simulink model "DTNS_SIM2"  (R2022a)
settings: Solver=ode4  StartTime=0.0  StopTime=100  FixedStep=0.01  RelTol=1e-3  EnableMultiTasking=on
PreLoadFcn:
  | listing = dir;
  | if (contains([listing.name], 'MAP')) &&  (contains([listing.name], 'DTNS_SIM.slx'))
  |     addpath('./AGR', './TRN', './TCAF', './FTG', './DYN', './FLCC', './GPS', './RALT', './INS', './MAP');
  |     addpath('./MAP/MAP_DB');
  | else
  |     warning('[DTNS_SIM.slx]는 DTNS 프로젝트 최상단 경로에 위치해야 합니다.');
  | end
  | 
  | load('BUS_STRUCTURE_DYN.mat');
  | load('BUS_STRUCTURE_FLCC.mat');
  | load('BUS_STRUCTURE_RALT.mat');
  | load('BUS_STRUCTURE_INS.mat');
  | load('BUS_STRUCTURE_GPS.mat');
  | load('BusStructureTRN.mat');
  | load('BusStructureLOSR.mat');
  | load('BusStructureHR.mat');
  | load('BusStructureCR.mat');
  | FTG_initState;
InitFcn:
  | listing = dir;
  | if (contains([listing.name], 'MAP')) &&  (contains([listing.name], 'DTNS_SIM.slx'))
  |     addpath('./AGR', './TRN', './TCAF', './FTG', './DYN', './FLCC', './GPS', './RALT', './INS', './MAP');
  |     addpath('./MAP/MAP_DB');
  | else
  |     warning('[DTNS_SIM.slx]는 DTNS 프로젝트 최상단 경로에 위치해야 합니다.');
  | end
  | 
  | load('BUS_STRUCTURE_DYN.mat');
  | load('BUS_STRUCTURE_FLCC.mat');
  | load('BUS_STRUCTURE_RALT.mat');
  | load('BUS_STRUCTURE_INS.mat');
  | load('BUS_STRUCTURE_GPS.mat');
  | load('BusStructureTRN.mat');
  | load('BusStructureLOSR.mat');
  | load('BusStructureHR.mat');
  | load('BusStructureCR.mat');
  | FTG_initState;
libraries: aerolibconvert2 x14, simulink_extras x5
(part 2 of 2)

== matlab function DTNS_SIM2/ControlTFInput ==
  data: inBus input Bus: DTFInput; DTFInput output Bus: DTFInput; RALTDatapumpPrev input
function DTFInput = ControlTFInput(inBus, RALTDatapumpPrev)
%ControlTFInput
persistent time dt
if isempty(time)
    time = 0.0;
end
if isempty(dt)
    dt = 0.01;
end
% -------------------------------------------------------------------------
% CONTROL flag
CONTROL_ACTIVATED = true;

% Copy
DTFInput = inBus;

if CONTROL_ACTIVATED
    % Default
    DTFInput.selected   = SET_VALUE(DTFInput.selected, true, time, 0, inf);
    DTFInput.rideQuality= SET_VALUE(DTFInput.rideQuality, uint16(3), time, 0, inf);
    DTFInput.msd        = SET_VALUE(DTFInput.msd, 500, time, 0, inf);
    DTFInput.raltValid  = SET_VALUE(DTFInput.raltValid, RALTDatapumpPrev.RadarAltitudeValid, time, 0, inf);
    DTFInput.raltAlt    = SET_VALUE(DTFInput.raltAlt, RALTDatapumpPrev.RadarAltitude, time, 0, inf);

    % Control
%     outBus.msd = SET_VALUE(outBus.msd, 500, time, 100, 50);
%     outBus.msd = SET_VALUE(outBus.msd, 500, time, 200, 50);

end

% Update Time
time = time + dt;
end

function out = SET_VALUE(in, value, curTime, triggerTime, duration)
out = in;
if (triggerTime <= curTime) && (curTime <= triggerTime+duration)
    out = value;
else
end
end

== matlab function DTNS_SIM2/TRNDataProcess/Subsystem3/Flag_WoW ==
  data: time input; WeightOnWheels output
function WeightOnWheels  = fcn(time)

% WeightOnWheels
% False[0]_flight / True[1]_ground

% if time <= 30
if time < 0
    WeightOnWheels = boolean(true);
else
    WeightOnWheels = boolean(false);
end

end

== matlab function DTNS_SIM2/TRNDataProcess/Subsystem3/MATLAB Function ==
  data: count input; count output
function count = fcn(count)

count = count + 0.04;

== matlab function DTNS_SIM2/TRNDataProcess/Subsystem3/Subsystem1/MATLAB Function1 ==
  data: WoW input; time input; lat_bias output; lon_bias output
function [lat_bias,lon_bias] = fcn(WoW, time)
%% parameters
lat2m = 111000;
lon2m = 91170;
bias1 = 200;   % 500m
bias2 = 200;   % 500m


%%
% if time > 60
if time >= 0
    if WoW == 0                % 0_flight / 1_ground
        lat_bias = bias1/lat2m;
        lon_bias = bias2/lon2m;
    else
        lat_bias = 0;
        lon_bias = 0;
    end
else
    lat_bias = 0;
    lon_bias = 0;
end

== matlab function DTNS_SIM2/TRNDataProcess/Subsystem3/Subsystem1/MATLAB Function3 ==
  data: u input; a output; b output
function [a,b]  = fcn(u)

% WeightOnWheels
if(u==1)
    a = boolean(true);
    b = boolean(true);
else
    a = boolean(false);
    b = boolean(false);
end

end

== matlab function DTNS_SIM2/Visualize/calcTerrainRoughness ==
  data: lat input; R output; lon input; hDEM output
function [R, hDEM] = calcTerrainRoughness(lat, lon)

lat2m = 110961.7060516;
lon2m = 89476.51124;

d_Lat = 90/lat2m; d_Lon = 90/lon2m;
d = 90;

hDEM = 0.0;
A=0.0; B=0.0; C=0.0; D=0.0; E=0.0; F=0.0; G=0.0; H=0.0; I=0.0; 

A = coder.ceval('MAPGetTerrainHeight', lat+d_Lat, lon-d_Lon);
B = coder.ceval('MAPGetTerrainHeight', lat+d_Lat, lon);
C = coder.ceval('MAPGetTerrainHeight', lat+d_Lat, lon+d_Lon);
D = coder.ceval('MAPGetTerrainHeight', lat, lon-d_Lon);
E = coder.ceval('MAPGetTerrainHeight', lat, lon);
F = coder.ceval('MAPGetTerrainHeight', lat, lon+d_Lon);
G = coder.ceval('MAPGetTerrainHeight', lat-d_Lat, lon-d_Lon);
H = coder.ceval('MAPGetTerrainHeight', lat-d_Lat, lon);
I = coder.ceval('MAPGetTerrainHeight', lat-d_Lat, lon+d_Lon);

SLP_CR=((C+F+I)-(A+D+G))/(6*d);
SLP_DR=((A+B+C)-(G+H+I))/(6*d);

mean_R=((mean(SLP_CR)-mean(SLP_DR))/2)^2;
std_R=((std(SLP_CR)^2)+(std(SLP_DR)^2))/2;

R=sqrt(mean_R+std_R)*100;

hDEM = E;

end
